simulink model "ANC_try3"  (R2016b)
settings: Solver=VariableStepAuto  StartTime=0.0  StopTime=10.0  RelTol=1e-3
libraries: dspvision x1, audiosources x1, dspadpt3 x1, dspobslib x1
settings Model: Creator=Ernest  LastModifiedBy=Ernest

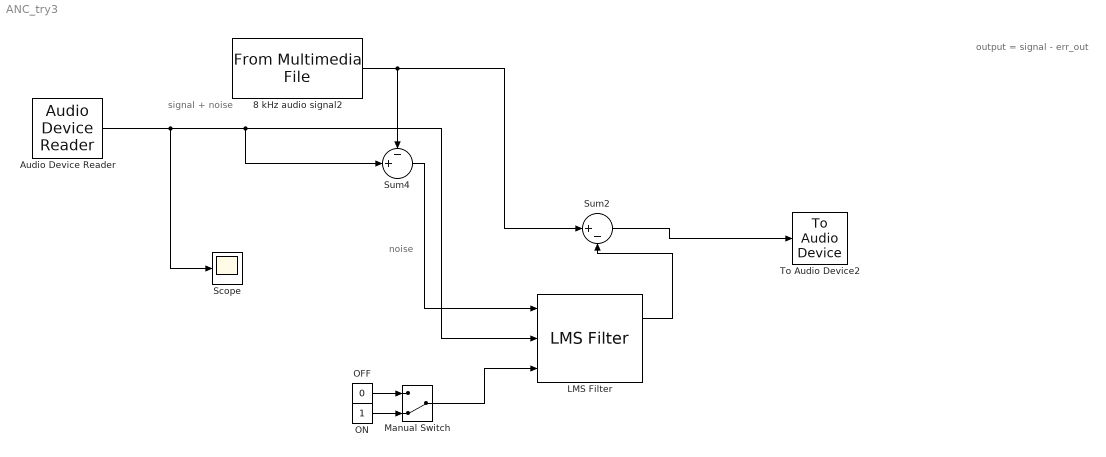
== system ANC_try3 ==
  note: output = signal - err_out
  note: noise
  note: signal + noise
  8 kHz audio signal2 : dspvision/From Multimedia File  inputFilename=/Projects/SS_proj/SigalChannelLiberation.wav  loop=on  numPlays=inf  outputStreams=Audio only  videoDataType=single  audioDataType=single  inheritSampleTime=on  userDefinedSampleTime=1/250  noAudioOutput=off  isIntensityVideo=off  fourcc=RGB  colorVideoFormat=Separate color signals  outputEOF=off  dataOrg=Column-major  audioFrameSize=32  computeAudioFrameSize=off  outSamplingMode=Sample based
  Audio Device Reader : audiosources/Audio Device Reader  Driver=CoreAudio  Device=Default  SampleRate=44100  NumChannels=1  SamplesPerFrame=32  BitDepth=16-bit integer  NumBuffers=10  DefaultInputChannelMapping=on  InputChannelMapping=1:2  OutputNumOverrunSamples=off  OutputDataType=double  DriverIdx=5  DeviceWarnFlag=''
  LMS Filter : dspadpt3/LMS Filter  Algo=LMS  L=32  stepflag=Dialog  mu=0.0008  leakage=1.0  ic=0  Adapt=on  resetflag=None  weights=off  secondCoeffMode=User-defined  secondCoeffWordLength=2  secondCoeffFracLength=15  accum2Mode=User-defined  accum2FracLength=20  prodOutput2Mode=User-defined  prodOutput2FracLength=20  prodOutput3Mode=User-defined  prodOutput3FracLength=20  prodOutput4Mode=User-defined  prodOutput4FracLength=20  quotientMode=User-defined  quotientFracLength=20  roundingMode=Floor  overflowMode=off  addnparflag=off
  Manual Switch : ManualSwitch  CurrentSetting=0
  OFF : Constant  Value=0
  ON : Constant
  Scope : Scope
  Sum2 : Sum  Inputs=|+-
  Sum4 : Sum  Inputs=-+|
  To Audio Device2 : dspobslib/To Audio Device  deviceName=Primary Sound Driver  inheritSampleRate=on  sampleRate=44100  deviceDatatype=Determine from input data type  autoBufferSize=on  bufferSize=4096  queueDuration=1.0  defaultOutputChannelMapping=on  outputChannelMapping=1:2  outputNumUnderrunSamples=off
  wires:
  8 kHz audio signal2/1 -> Sum4/1, Sum2/1
  Audio Device Reader/1 -> Scope/1, Sum4/2, LMS Filter/2
  OFF/1 -> Manual Switch/1
  ON/1 -> Manual Switch/2
  Manual Switch/1 -> LMS Filter/3
  Sum2/1 -> To Audio Device2/1
  LMS Filter/1 -> Sum2/2
  Sum4/1 -> LMS Filter/1
